simulink model "Pub_Sensor_20180704"  (R2018a)
settings: Solver=VariableStepAuto  StartTime=0.0  StopTime=inf  RelTol=1e-3
undefined symbols (not defined in the file or in its folder): D, DiscIntNeverNeededParam, G, serial, Twist
libraries: xpcutilitieslib x20, instrumentlib x9, robotlib x4, commutil2 x2, dsparch4 x1, simulink x1
settings Model: Creator=Nishida-Lab  LastModifiedBy=Nishida-Lab

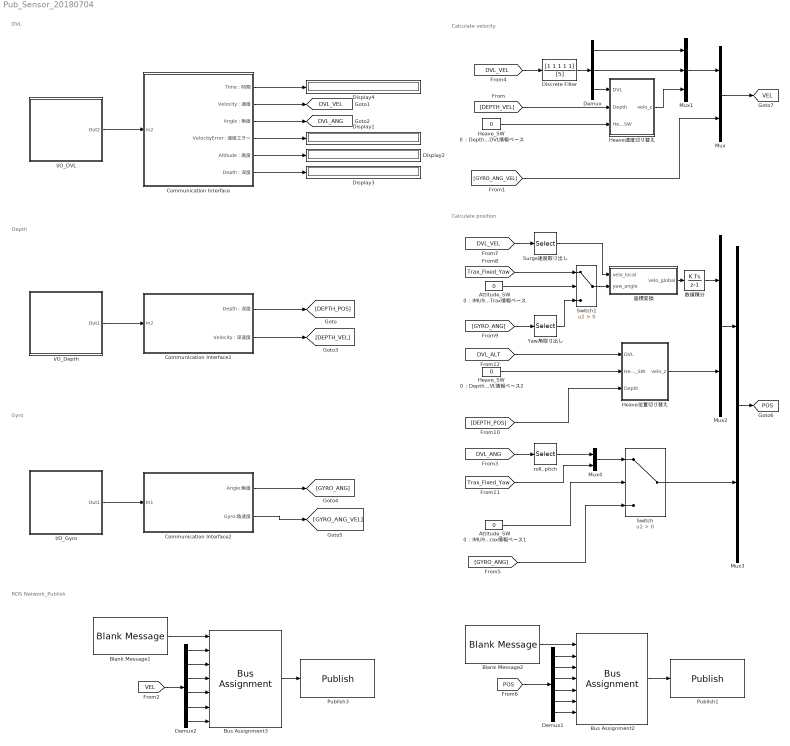
== system Pub_Sensor_20180704 ==
  note: ROS Network_Publish
  note: Gyro
  note: Depth
  note: DVL
  note: Calculate velocity
  note: Calculate position
  Attitude_SW ０：IMU9250情報ベース １：Trax情報ベース : Constant  Value=0
  Attitude_SW ０：IMU9250情報ベース １：Trax情報ベース1 : Constant  Value=0
  Blank Message1 : robotlib/Blank Message  SourceLibraryInfo=This block requires Robotics System Toolbox  messageType=geometry_msgs/TwistStamped  SampleTime=inf
      settings: SourceProductBaseCode=RO
  Blank Message2 : robotlib/Blank Message  SourceLibraryInfo=This block requires Robotics System Toolbox  messageType=geometry_msgs/TwistStamped  SampleTime=inf
      settings: SourceProductBaseCode=RO
  Bus Assignment2 : BusAssignment  AssignedSignals=Twist.Linear.X,Twist.Linear.Y,Twist.Linear.Z,Twist.Angular.X,Twist.Angular.Y,Twist.Angular.Z
  Bus Assignment3 : BusAssignment  AssignedSignals=Twist.Linear.X,Twist.Linear.Y,Twist.Linear.Z,Twist.Angular.X,Twist.Angular.Y,Twist.Angular.Z
  Communication Interface : Subsystem
  Communication Interface1 : Subsystem
  Communication Interface2 : Subsystem
  Demux : Demux  Outputs=3
  Demux1 : Demux  Outputs=6
  Demux2 : Demux  Outputs=6
  Discrete Filter : DiscreteFilter  Numerator=[1 1 1 1 1]  Denominator=[5]
  Display{1..4} (4 alike) : Display
  Heave_SW ０：Depth情報ベース １：DVL情報ベース : Constant  Value=0
  Heave_SW ０：Depth情報ベース １：DVL情報ベース2 : Constant  Value=0
  Heave位置切り替え : Subsystem
  Heave速度切り替え : Subsystem
  I/O_DVL : Subsystem
  I/O_Depth : Subsystem
  I/O_Gyro : Subsystem
  Mux{,2..4} (4 alike) : Mux  Inputs=2
  Mux1 : Mux  Inputs=3
  Publish1 : robotlib/Publish  SourceLibraryInfo=This block requires Robotics System Toolbox  topicSource=Specify your own  topic=/RT_POS  messageType=geometry_msgs/TwistStamped  messageQueueLength=1
      settings: SourceProductBaseCode=RO
  Publish3 : robotlib/Publish  SourceLibraryInfo=This block requires Robotics System Toolbox  topicSource=Specify your own  topic=/RT_VEL  messageType=geometry_msgs/TwistStamped  messageQueueLength=1
      settings: SourceProductBaseCode=RO
  Surge速度取り出し : Selector  InputPortWidth=3  IndexOptions=Index vector (dialog)  Indices=[1 2]  OutputSizes=1
  Switch : Switch  Criteria=u2 > Threshold
  Switch1 : Switch  Criteria=u2 > Threshold
  Yaw角取り出し : Selector  InputPortWidth=3  IndexOptions=Index vector (dialog)  Indices=[3]  OutputSizes=1
  "roll, pitch" : Selector  InputPortWidth=3  IndexOptions=Index vector (dialog)  Indices=[1 2]  OutputSizes=1
  座標変換 : MATLAB Function  TreatAsAtomicUnit=on
  数値積分 : DiscreteIntegrator  InitialCondition=[0 ; 0]  SampleTime=-1  ICPrevOutput=DiscIntNeverNeededParam  ICPrevScaledInput=DiscIntNeverNeededParam
  tag scope: DVL_ANG=global, DVL_VEL=global, POS=global, VEL=global
  wires:
  I/O_Depth/1(Out1) -> Communication Interface1/1(In2)
  I/O_DVL/1(Out2) -> Communication Interface/1(In2)
  Communication Interface/1(Time：時間) -> Display4/1
  Communication Interface/2(Velocity：速度) -> [DVL_VEL]
  Communication Interface/3("Angle : 角度") -> [DVL_ANG]
  Communication Interface/4(VelocityError：速度エラー) -> Display1/1
  Communication Interface/5(Altitude：高度) -> Display2/1
  Communication Interface/6(Depth：深度) -> Display3/1
  Communication Interface1/2(Velocity：深速度) -> [DEPTH_VEL]
  Communication Interface1/1(Depth：深度) -> [DEPTH_POS]
  I/O_Gyro/1(Out1) -> Communication Interface2/1(In1)
  Communication Interface2/1(Angle:角度) -> [GYRO_ANG]
  Communication Interface2/2(Gyro:角速度) -> [GYRO_ANG_VEL]
  Heave_SW ０：Depth情報ベース １：DVL情報ベース2/1 -> Heave位置切り替え/2(Heave_SW)
  [Trax_Fixed_Yaw] -> Switch1/1
  Heave速度切り替え/1(velo_z) -> Mux1/3
  Yaw角取り出し/1 -> Switch1/3
  [GYRO_ANG] -> Switch/3
  [DEPTH_POS] -> Heave位置切り替え/3(Depth)
  Heave位置切り替え/1(velo_z) -> Mux2/2
  [GYRO_ANG] -> Yaw角取り出し/1
  Mux3/1 -> [POS]
  Switch1/1 -> 座標変換/2(yaw_angle)
  [DVL_ALT] -> Heave位置切り替え/1(DVL)
  座標変換/1(velo_global) -> 数値積分/1
  Mux2/1 -> Mux3/1
  Attitude_SW ０：IMU9250情報ベース １：Trax情報ベース1/1 -> Switch/2
  "roll, pitch"/1 -> Mux4/1
  Demux/2 -> Mux1/2
  数値積分/1 -> Mux2/1
  [DVL_VEL] -> Surge速度取り出し/1
  [Trax_Fixed_Yaw] -> Mux4/2
  Attitude_SW ０：IMU9250情報ベース １：Trax情報ベース/1 -> Switch1/2
  Mux/1 -> [VEL]
  Mux1/1 -> Mux/1
  [DVL_ANG] -> "roll, pitch"/1
  Switch/1 -> Mux3/2
  Discrete Filter/1 -> Demux/1
  Demux/1 -> Mux1/1
  Surge速度取り出し/1 -> 座標変換/1(velo_local)
  Heave_SW ０：Depth情報ベース １：DVL情報ベース/1 -> Heave速度切り替え/3(HeaveSW)
  Demux/3 -> Heave速度切り替え/1(DVL)
  [GYRO_ANG_VEL] -> Mux/2
  [DEPTH_VEL] -> Heave速度切り替え/2(Depth)
  [DVL_VEL] -> Discrete Filter/1
  Mux4/1 -> Switch/1
  Bus Assignment3/1 -> Publish3/1
  Demux2/3 -> Bus Assignment3/4
  [VEL] -> Demux2/1
  Demux2/2 -> Bus Assignment3/3
  Demux2/4 -> Bus Assignment3/5
  Demux2/6 -> Bus Assignment3/7
  Demux2/5 -> Bus Assignment3/6
  Blank Message1/1 -> Bus Assignment3/1
  Demux2/1 -> Bus Assignment3/2
  Demux1/1 -> Bus Assignment2/2
  [POS] -> Demux1/1
  Demux1/3 -> Bus Assignment2/4
  Demux1/6 -> Bus Assignment2/7
  Demux1/2 -> Bus Assignment2/3
  Blank Message2/1 -> Bus Assignment2/1
  Demux1/4 -> Bus Assignment2/5
  Bus Assignment2/1 -> Publish1/1
  Demux1/5 -> Bus Assignment2/6

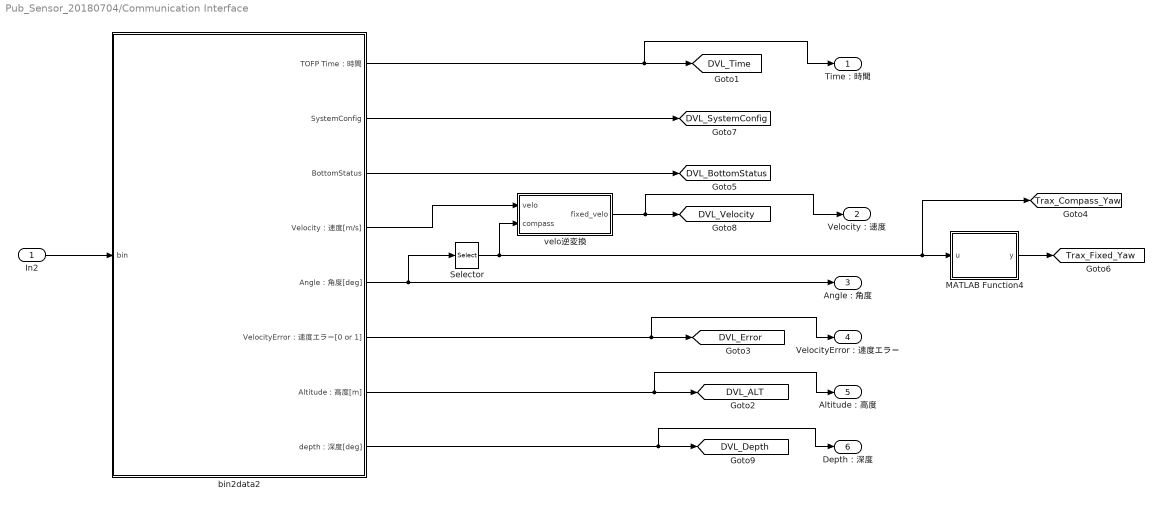
== system Pub_Sensor_20180704/Communication Interface ==
  In2 : Inport
  MATLAB Function4 : MATLAB Function  TreatAsAtomicUnit=on
  Selector : Selector  InputPortWidth=3  IndexOptions=Index vector (dialog)  Indices=[3]  OutputSizes=1
  bin2data2 : Subsystem
  velo逆変換 : Subsystem
  Time：時間 : Outport
  Velocity：速度 : Outport  Port=2
  "Angle : 角度" : Outport  Port=3
  VelocityError：速度エラー : Outport  Port=4
  Altitude：高度 : Outport  Port=5
  Depth：深度 : Outport  Port=6
  tag scope: DVL_ALT=global, DVL_BottomStatus=global, DVL_Depth=global, DVL_Error=global, DVL_SystemConfig=global, DVL_Time=global, DVL_Velocity=global, Trax_Compass_Yaw=global, Trax_Fixed_Yaw=global
  wires:
  velo逆変換/1(fixed_velo) -> Velocity：速度/1, [DVL_Velocity]
  bin2data2/5(Angle：角度[deg]) -> Selector/1, "Angle : 角度"/1
  bin2data2/3(BottomStatus) -> [DVL_BottomStatus]
  bin2data2/8(depth：深度[deg]) -> Depth：深度/1, [DVL_Depth]
  In2/1 -> bin2data2/1(bin)
  MATLAB Function4/1(y) -> [Trax_Fixed_Yaw]
  bin2data2/7(Altitude：高度[m]) -> [DVL_ALT], Altitude：高度/1
  bin2data2/6(VelocityError：速度エラー[0 or 1]) -> [DVL_Error], VelocityError：速度エラー/1
  bin2data2/1(TOFP Time：時間) -> Time：時間/1, [DVL_Time]
  bin2data2/2(SystemConfig) -> [DVL_SystemConfig]
  bin2data2/4(Velocity：速度[m/s]) -> velo逆変換/1(velo)
  Selector/1 -> [Trax_Compass_Yaw], MATLAB Function4/1(u), velo逆変換/2(compass)

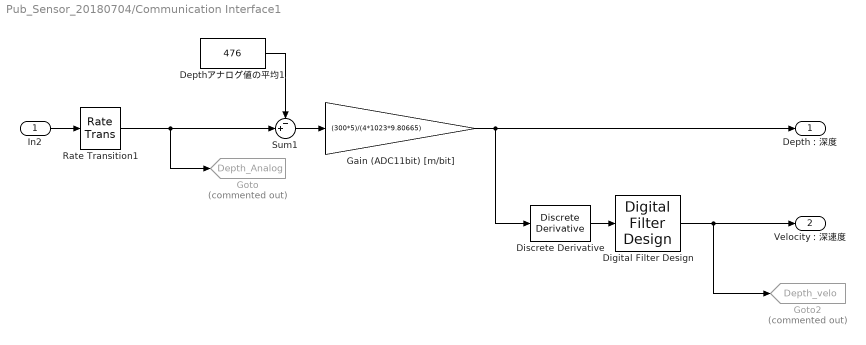
== system Pub_Sensor_20180704/Communication Interface1 ==
  In2 : Inport
  Depthアナログ値の平均1 : Constant  Value=476
  Digital Filter Design : dsparch4/Digital Filter Design  mwdsp_browser_bugfix_var=off
  Discrete Derivative : simulink/Discrete/Discrete Derivative  gainval=1.0  ICPrevScaledInput=0.0  InputProcessing=Inherited  OutMin=[]  OutMax=[]  OutDataType=fixdt(1, 16)  OutScaling=2^-10  DoSatur=off
  Gain (ADC11bit) [m/bit] : Gain  Gain=(300*5)/(4*1023*9.80665)
  Goto : Goto  Commented=on  GotoTag=Depth_Analog  TagVisibility=global
  Goto2 : Goto  Commented=on  GotoTag=Depth_velo  TagVisibility=global
  Rate Transition1 : RateTransition  OutPortSampleTime=0.1
  Sum1 : Sum  Inputs=-+|
  Depth：深度 : Outport
  Velocity：深速度 : Outport  Port=2
  wires:
  Digital Filter Design/1 -> Goto2/1, Velocity：深速度/1
  In2/1 -> Rate Transition1/1
  Gain (ADC11bit) [m/bit]/1 -> Discrete Derivative/1, Depth：深度/1
  Sum1/1 -> Gain (ADC11bit) [m/bit]/1
  Depthアナログ値の平均1/1 -> Sum1/1
  Rate Transition1/1 -> Goto/1, Sum1/2
  Discrete Derivative/1 -> Digital Filter Design/1

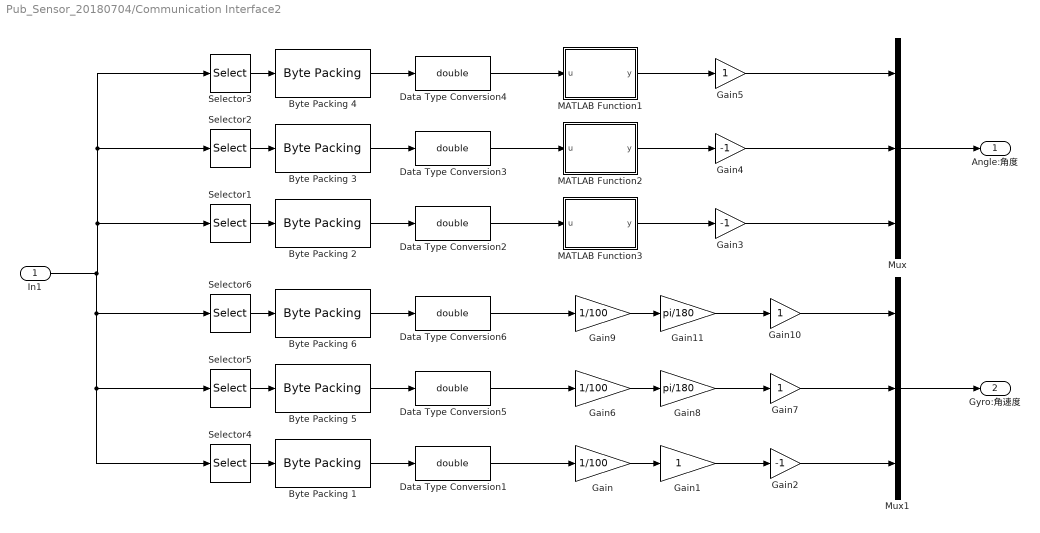
== system Pub_Sensor_20180704/Communication Interface2 ==
  In1 : Inport
  Byte Packing {1..6} (6 alike) : xpcutilitieslib/Byte Packing 
  Data Type Conversion{1..6} (6 alike) : DataTypeConversion  OutDataTypeStr=double
  Gain : Gain  Gain=1/100
  Gain{1,5,7,10} (4 alike) : Gain
  Gain11 : Gain  Gain=pi/180
  Gain2 : Gain  Gain=-1
  Gain3 : Gain  Gain=-1
  Gain4 : Gain  Gain=-1
  Gain6 : Gain  Gain=1/100
  Gain8 : Gain  Gain=pi/180
  Gain9 : Gain  Gain=1/100
  MATLAB Function1 : MATLAB Function  TreatAsAtomicUnit=on
  MATLAB Function2 : MATLAB Function  TreatAsAtomicUnit=on
  MATLAB Function3 : MATLAB Function  TreatAsAtomicUnit=on
  Mux : Mux  Inputs=3
  Mux1 : Mux  Inputs=3
  Selector1 : Selector  InputPortWidth=12  IndexOptions=Index vector (dialog)  Indices=[2 1]  OutputSizes=1
  Selector2 : Selector  InputPortWidth=12  IndexOptions=Index vector (dialog)  Indices=[4 3]  OutputSizes=1
  Selector3 : Selector  InputPortWidth=12  IndexOptions=Index vector (dialog)  Indices=[6 5]  OutputSizes=1
  Selector4 : Selector  InputPortWidth=12  IndexOptions=Index vector (dialog)  Indices=[8 7]  OutputSizes=1
  Selector5 : Selector  InputPortWidth=12  IndexOptions=Index vector (dialog)  Indices=[10 9]  OutputSizes=1
  Selector6 : Selector  InputPortWidth=12  IndexOptions=Index vector (dialog)  Indices=[12 11]  OutputSizes=1
  Angle:角度 : Outport
  Gyro:角速度 : Outport  Port=2
  wires:
  In1/1 -> Selector2/1, Selector3/1, Selector1/1, Selector4/1, Selector5/1, Selector6/1
  Gain/1 -> Gain1/1
  Byte Packing 1/1 -> Data Type Conversion1/1
  MATLAB Function3/1(y) -> Gain3/1
  Data Type Conversion4/1 -> MATLAB Function1/1(u)
  Gain3/1 -> Mux/3
  Selector6/1 -> Byte Packing 6/1
  Selector2/1 -> Byte Packing 3/1
  Gain6/1 -> Gain8/1
  MATLAB Function2/1(y) -> Gain4/1
  Gain8/1 -> Gain7/1
  Data Type Conversion1/1 -> Gain/1
  Selector4/1 -> Byte Packing 1/1
  Gain4/1 -> Mux/2
  Gain2/1 -> Mux1/3
  Selector3/1 -> Byte Packing 4/1
  Data Type Conversion5/1 -> Gain6/1
  Data Type Conversion3/1 -> MATLAB Function2/1(u)
  Gain10/1 -> Mux1/1
  Data Type Conversion6/1 -> Gain9/1
  Byte Packing 5/1 -> Data Type Conversion5/1
  Gain9/1 -> Gain11/1
  Gain5/1 -> Mux/1
  Gain11/1 -> Gain10/1
  Data Type Conversion2/1 -> MATLAB Function3/1(u)
  Byte Packing 6/1 -> Data Type Conversion6/1
  MATLAB Function1/1(y) -> Gain5/1
  Gain7/1 -> Mux1/2
  Mux/1 -> Angle:角度/1
  Gain1/1 -> Gain2/1
  Byte Packing 3/1 -> Data Type Conversion3/1
  Byte Packing 2/1 -> Data Type Conversion2/1
  Byte Packing 4/1 -> Data Type Conversion4/1
  Selector5/1 -> Byte Packing 5/1
  Mux1/1 -> Gyro:角速度/1
  Selector1/1 -> Byte Packing 2/1

== system Pub_Sensor_20180704/Heave位置切り替え ==
  DVL : Inport
  Heave_SW : Inport  Port=2
  Depth : Inport  Port=3
  Switch : Switch  Criteria=u2 > Threshold
  velo_z : Outport
  wires:
  Depth/1 -> Switch/3
  DVL/1 -> Switch/1
  Heave_SW/1 -> Switch/2
  Switch/1 -> velo_z/1

== system Pub_Sensor_20180704/Heave速度切り替え ==
  DVL : Inport
  Depth : Inport  Port=2
  HeaveSW : Inport  Port=3
  Switch : Switch  Criteria=u2 > Threshold
  velo_z : Outport
  wires:
  Depth/1 -> Switch/3
  DVL/1 -> Switch/1
  HeaveSW/1 -> Switch/2
  Switch/1 -> velo_z/1

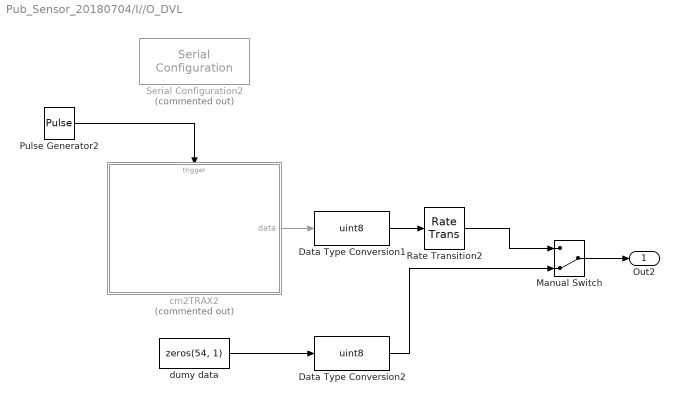
== system Pub_Sensor_20180704/I//O_DVL ==
  Data Type Conversion1 : DataTypeConversion  OutDataTypeStr=uint8
  Data Type Conversion2 : DataTypeConversion  OutDataTypeStr=uint8
  Manual Switch : ManualSwitch  CurrentSetting=0
  Pulse Generator2 : DiscretePulseGenerator  PulseType=Time based  Period=0.2  PulseWidth=50
  Rate Transition2 : RateTransition  OutPortSampleTime=0.1
  Serial Configuration2 : instrumentlib/Serial Configuration  Priority=-200000  Commented=on  ComPortMenu=<Please select a port...>  ComPort=COM7  ObjConstructor=serial('COM7');  BaudRate=115200  DataBits=8  Parity=none  StopBits=1  FlowControl=none  Timeout=10  ByteOrder=LittleEndian
  cm2TRAX2 : Stateflow chart  Commented=on  TreatAsAtomicUnit=on
  dumy data : Constant  Value=zeros(54, 1)
  Out2 : Outport
  wires:
  cm2TRAX2/1(data) -> Data Type Conversion1/1
  Data Type Conversion2/1 -> Manual Switch/2
  Rate Transition2/1 -> Manual Switch/1
  Data Type Conversion1/1 -> Rate Transition2/1
  Manual Switch/1 -> Out2/1
  dumy data/1 -> Data Type Conversion2/1
  Pulse Generator2/1 -> cm2TRAX2/Trigger

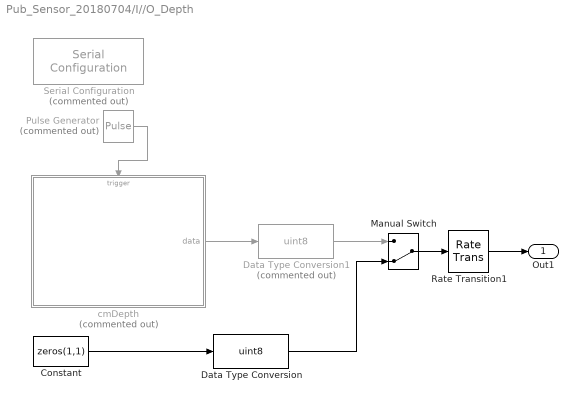
== system Pub_Sensor_20180704/I//O_Depth ==
  Constant : Constant  Value=zeros(1,1)  VectorParams1D=off
  Data Type Conversion : DataTypeConversion  OutDataTypeStr=uint8
  Data Type Conversion1 : DataTypeConversion  Commented=on  OutDataTypeStr=uint8
  Manual Switch : ManualSwitch  CurrentSetting=0
  Pulse Generator : DiscretePulseGenerator  Commented=on  PulseType=Time based  Period=0.1  PulseWidth=50
  Rate Transition1 : RateTransition  OutPortSampleTime=0.1
  Serial Configuration : instrumentlib/Serial Configuration  Priority=-200000  Commented=on  ComPortMenu=<Please select a port...>  ComPort=COM21  ObjConstructor=serial('COM21');  BaudRate=115200  DataBits=8  Parity=none  StopBits=1  FlowControl=none  Timeout=10  ByteOrder=LittleEndian
  cmDepth : Stateflow chart  Commented=on  TreatAsAtomicUnit=on
  Out1 : Outport
  wires:
  Pulse Generator/1 -> cmDepth/Trigger
  Constant/1 -> Data Type Conversion/1
  Data Type Conversion/1 -> Manual Switch/2
  Manual Switch/1 -> Rate Transition1/1
  Rate Transition1/1 -> Out1/1
  Data Type Conversion1/1 -> Manual Switch/1
  cmDepth/1(data) -> Data Type Conversion1/1

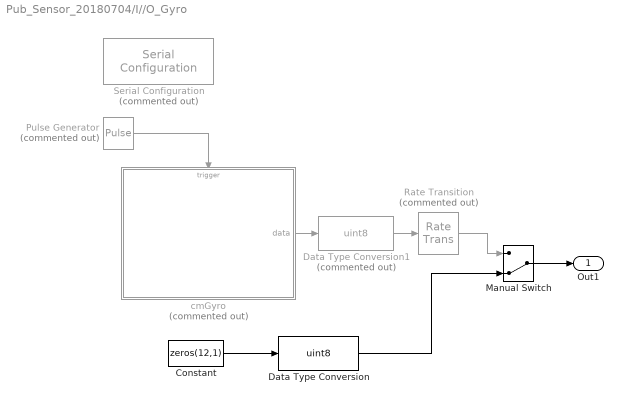
== system Pub_Sensor_20180704/I//O_Gyro ==
  Constant : Constant  Value=zeros(12,1)
  Data Type Conversion : DataTypeConversion  OutDataTypeStr=uint8
  Data Type Conversion1 : DataTypeConversion  Commented=on  OutDataTypeStr=uint8
  Manual Switch : ManualSwitch  CurrentSetting=0
  Pulse Generator : DiscretePulseGenerator  Commented=on  PulseType=Time based  Period=0.1  PulseWidth=50
  Rate Transition : RateTransition  Commented=on  OutPortSampleTime=0.1
  Serial Configuration : instrumentlib/Serial Configuration  Priority=-200000  Commented=on  ComPortMenu=<Please select a port...>  ComPort=COM14  ObjConstructor=serial('COM14');  BaudRate=115200  DataBits=8  Parity=none  StopBits=1  FlowControl=none  Timeout=10  ByteOrder=LittleEndian
  cmGyro : Stateflow chart  Commented=on  TreatAsAtomicUnit=on
  Out1 : Outport
  wires:
  cmGyro/1(data) -> Data Type Conversion1/1
  Pulse Generator/1 -> cmGyro/Trigger
  Data Type Conversion1/1 -> Rate Transition/1
  Data Type Conversion/1 -> Manual Switch/2
  Manual Switch/1 -> Out1/1
  Constant/1 -> Data Type Conversion/1
  Rate Transition/1 -> Manual Switch/1

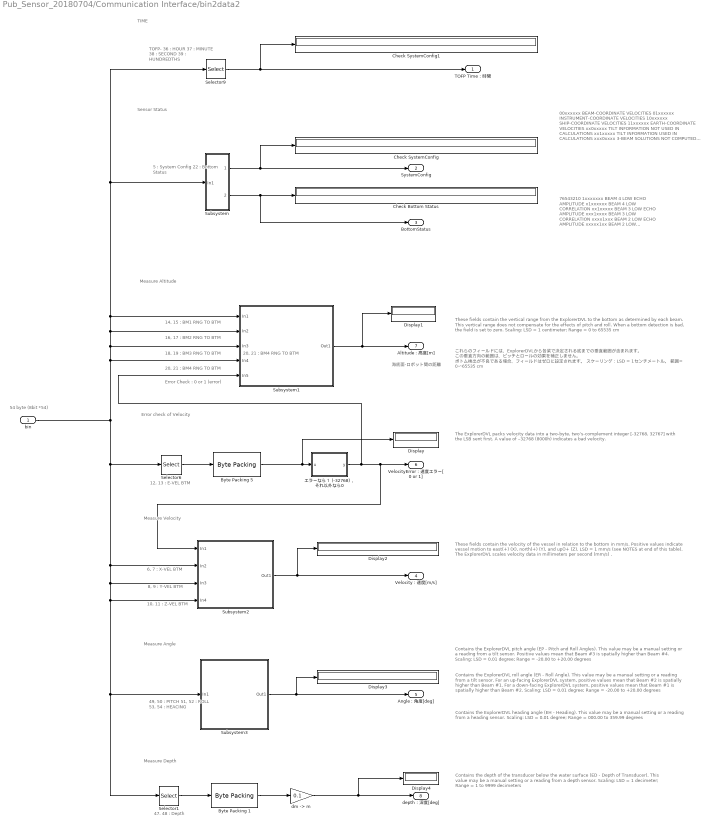
== system Pub_Sensor_20180704/Communication Interface/bin2data2 ==
  note: Contains the depth of the transducer below the water surface (ED - Depth of Transducer).
      | This value may be a manual setting or a reading from a depth sensor.
      | Scaling: LSD = 1 decimeter; Range = 1 to 9999 decimeters
  note: 54 byte (8bit *54)
  note: Contains the ExplorerDVL heading angle (EH - Heading). This value may be a manual setting or a reading from a heading sensor.
      | Scaling: LSD = 0.01 degree; Range = 000.00 to 359.99 degrees
  note: Contains the ExplorerDVL roll angle (ER - Roll Angle). This value may be a manual setting or a reading from a tilt sensor. For an up-facing ExplorerDVL system, positive values mean that Beam #2 is spatially higher than Beam #1. For a down-facing ExplorerDVL system, positive values mean that Beam #1 is spatially higher than Beam #2.
      | Scaling: LSD = 0.01 degree; Range = -20.00 to +20.00 degrees
  note: Contains the ExplorerDVL pitch angle (EP - Pitch and Roll Angles). This value may be a manual setting or a reading from a tilt sensor. Positive values mean that Beam #3 is spatially higher than Beam #4.
      | Scaling: LSD = 0.01 degree; Range = -20.00 to +20.00 degrees
  note: The ExplorerDVL packs velocity data into a two-byte, two’s-complement integer [-32768, 32767]
      | with the LSB sent first.
      | A value of –32768 (8000h) indicates a bad velocity.
  note: These fields contain the velocity of the vessel in relation to the bottom in mm/s. Positive
      | values indicate vessel motion to east(+) (X), north(+) (Y), and up()+ (Z). LSD = 1 mm/s (see NOTES at
      | end of this table).
      | The ExplorerDVL scales velocity data in millimeters per second (mm/s) .
  note: これらのフィールドには、ExplorerDVLから各梁で決定される底までの垂直範囲が含まれます。
      | この垂直方向の範囲は、ピッチとロールの効果を補正しません。
      | ボトム検出が不良である場合、フィールドはゼロに設定されます。
      | スケーリング：LSD = 1センチメートル。 範囲= 0〜65535 cm
  note: 海底面-ロボット間の距離
  note: These fields contain the vertical range from the ExplorerDVL to the bottom as determined by each beam.
      | This vertical range does not compensate for the effects of pitch and roll.
      | When a bottom detection is bad, the field is set to zero.
      | Scaling: LSD = 1 centimeter; Range = 0 to 65535 cm
  note: Measure Altitude
  note: 5 : System Config
      | 22 : Bottom Status
  note: 76543210
      | 1xxxxxxx BEAM 4 LOW ECHO AMPLITUDE
      | x1xxxxxx BEAM 4 LOW CORRELATION
      | xx1xxxxx BEAM 3 LOW ECHO AMPLITUDE
      | xxx1xxxx BEAM 3 LOW CORRELATION
      | xxxx1xxx BEAM 2 LOW ECHO AMPLITUDE
      | xxxxx1xx BEAM 2 LOW CORRELATION
      | xxxxxx1x BEAM 1 LOW ECHO AMPLITUDE
      | xxxxxxx1 BEAM 1 LOW CORRELATION
  note: 00xxxxxx BEAM-COORDINATE VELOCITIES
      | 01xxxxxx INSTRUMENT-COORDINATE VELOCITIES
      | 10xxxxxx SHIP-COORDINATE VELOCITIES
      | 11xxxxxx EARTH-COORDINATE VELOCITIES
      | xx0xxxxx TILT INFORMATION NOT USED IN CALCULATIONS
      | xx1xxxxx TILT INFORMATION USED IN CALCULATIONS
      | xxx0xxxx 3-BEAM SOLUTIONS NOT COMPUTED
      | xxx1xxxx 3-BEAM SOLUTIONS COMPUTED
      | xxxxx001 150-kHz ExplorerDVL
      | xxxxx010 300-kHz ExplorerDVL
      | xxxxx011 600-kHz ExplorerDVL
      | xxxxx100 1200-kHz ExplorerDVL
  note: TIME
  note: 12, 13 : E-VEL BTM
  note: TOFP-
      | 36 : HOUR
      | 37 : MINUTE
      | 38 : SECOND
      | 39 : HUNDREDTHS
  note: Sensor Status
  note: 14, 15 : BM1 RNG TO BTM
  note: 16, 17 : BM2 RNG TO BTM
  note: 18, 19 : BM3 RNG TO BTM
  note: 20, 21 : BM4 RNG TO BTM
  note: 20, 21 : BM4 RNG TO BTM
  note: Error Check : 0 or 1 (error)
  note: Error check of Velocity
  note: Measure Velocity
  note: 6, 7 : X-VEL BTM
  note: 8, 9 : Y-VEL BTM
  note: 10, 11 : Z-VEL BTM
  note: 49, 50 : PITCH
      | 51, 52 : ROLL
      | 53, 54 : HEACING
  note: Measure Angle
  note: Measure Depth
  note: 47. 48 : Depth
  bin : Inport
  Byte Packing 1 : xpcutilitieslib/Byte Packing   MaskPackedDataType=int16  MaskUnpackedDataTypes={'uint8'}  MaskAlignment=2
  Byte Packing 5 : xpcutilitieslib/Byte Packing   MaskPackedDataType=int16  MaskUnpackedDataTypes={'uint8'}  MaskAlignment=2
  Check Bottom Status : Display
  Check SystemConfig : Display
  Check SystemConfig1 : Display
  Display{,1..4} (5 alike) : Display
  Selector1 : Selector  InputPortWidth=54  IndexOptions=Index vector (dialog)  Indices=[47 48]  OutputSizes=1
  Selector6 : Selector  InputPortWidth=54  IndexOptions=Index vector (dialog)  Indices=[12 13]  OutputSizes=1
  Selector9 : Selector  InputPortWidth=54  IndexOptions=Index vector (dialog)  Indices=[36 37 38 39]  OutputSizes=1
  Subsystem : Subsystem
  Subsystem1 : Subsystem
  Subsystem2 : Subsystem
  Subsystem3 : Subsystem
  "dm -> m" : Gain  Gain=0.1  OutDataTypeStr=double
  エラーなら１ (-32768)， それ以外なら0 : MATLAB Function  TreatAsAtomicUnit=on
  TOFP Time：時間 : Outport
  SystemConfig : Outport  Port=2
  BottomStatus : Outport  Port=3
  Velocity：速度[m/s] : Outport  Port=4
  Angle：角度[deg] : Outport  Port=5
  VelocityError：速度エラー[0 or 1] : Outport  Port=6
  Altitude：高度[m] : Outport  Port=7
  depth：深度[deg] : Outport  Port=8
  wires:
  Selector6/1 -> Byte Packing 5/1
  Byte Packing 5/1 -> Display/1, エラーなら１ (-32768)， それ以外なら0/1(u)
  Selector9/1 -> Check SystemConfig1/1, TOFP Time：時間/1
  エラーなら１ (-32768)， それ以外なら0/1(y) -> Subsystem1/5(In5), Subsystem2/1(In1), VelocityError：速度エラー[0 or 1]/1
  bin/1 -> Subsystem1/2(In2), Selector9/1, Subsystem/1(In1), Subsystem1/1(In1), Subsystem1/3(In3), Subsystem1/4(In4), Subsystem2/3(In3), Selector1/1, Subsystem3/1(In1), Subsystem2/4(In4), Subsystem2/2(In2), Selector6/1
  Subsystem/1(Out1) -> SystemConfig/1, Check SystemConfig/1
  Subsystem/2(Out2) -> BottomStatus/1, Check Bottom Status/1
  Subsystem1/1(Out1) -> Display1/1, Altitude：高度[m]/1
  Subsystem2/1(Out1) -> Display2/1, Velocity：速度[m/s]/1
  Subsystem3/1(Out1) -> Display3/1, Angle：角度[deg]/1
  Selector1/1 -> Byte Packing 1/1
  Byte Packing 1/1 -> "dm -> m"/1
  "dm -> m"/1 -> depth：深度[deg]/1, Display4/1

== system Pub_Sensor_20180704/Communication Interface/velo逆変換 ==
  velo : Inport
  compass : Inport  Port=2
  MATLAB Function : MATLAB Function  TreatAsAtomicUnit=on
  fixed_velo : Outport
  wires:
  velo/1 -> MATLAB Function/1(velo)
  compass/1 -> MATLAB Function/2(angle)
  MATLAB Function/1(y) -> fixed_velo/1

== system Pub_Sensor_20180704/I//O_DVL/cm2TRAX2/recieve.recieve_data ==
  f : TriggerPort  TriggerType=function-call  VariantControl=Variant
      settings: CopyFcn=Stateflow.SLINSF.SimulinkMan.removeBlockPreDeleteFcn  PreDeleteFcn=Stateflow.SLINSF.SimulinkMan.unsafePredeleteFcn
  Serial Receive : instrumentlib/Serial Receive  ComPortMenu=<Please select a port...>  ComPort=COM7  ObjConstructor=serial('COM7');  Header=CS<  Terminator=<none>  DataSize=54  DataType=uint8  EnableBlockingMode=off  ActionDataUnavailable=Output last received value  CustomValue=0  SampleTime=-1
  data : Outport  OutDataTypeStr=uint8  PortDimensions=54
  wires:
  Serial Receive/1 -> data/1

== system Pub_Sensor_20180704/I//O_DVL/cm2TRAX2/send.send_q ==
  f : TriggerPort  TriggerType=function-call  VariantControl=Variant
      settings: CopyFcn=Stateflow.SLINSF.SimulinkMan.removeBlockPreDeleteFcn  PreDeleteFcn=Stateflow.SLINSF.SimulinkMan.unsafePredeleteFcn
  Constant1 : Constant  Value=67  OutDataTypeStr=uint8
  Constant2 : Constant  Value=13  OutDataTypeStr=uint8
  Constant3 : Constant  Value=10  OutDataTypeStr=uint8
  Constant4 : Constant  Value=83  OutDataTypeStr=uint8
  Mux : Mux
  Serial Send : instrumentlib/Serial Send  ComPortMenu=<Please select a port...>  ComPort=COM7  ObjConstructor=serial('COM7');  Terminator=<none>  EnableBlockingMode=off
  wires:
  Mux/1 -> Serial Send/1
  Constant2/1 -> Mux/3
  Constant3/1 -> Mux/4
  Constant4/1 -> Mux/2
  Constant1/1 -> Mux/1

== system Pub_Sensor_20180704/I//O_Depth/cmDepth/recieve.recieve_data ==
  f : TriggerPort  TriggerType=function-call  VariantControl=Variant
      settings: CopyFcn=Stateflow.SLINSF.SimulinkMan.removeBlockPreDeleteFcn  PreDeleteFcn=Stateflow.SLINSF.SimulinkMan.unsafePredeleteFcn
  Serial Receive : instrumentlib/Serial Receive  ComPortMenu=<Please select a port...>  ComPort=COM21  ObjConstructor=serial('COM21');  Header=D:  Terminator=<none>  DataSize=1  DataType=int16  EnableBlockingMode=off  ActionDataUnavailable=Output last received value  CustomValue=0  SampleTime=-1
  data : Outport  OutDataTypeStr=int16  PortDimensions=1
  wires:
  Serial Receive/1 -> data/1

== system Pub_Sensor_20180704/I//O_Depth/cmDepth/send.send_q ==
  f : TriggerPort  TriggerType=function-call  VariantControl=Variant
      settings: CopyFcn=Stateflow.SLINSF.SimulinkMan.removeBlockPreDeleteFcn  PreDeleteFcn=Stateflow.SLINSF.SimulinkMan.unsafePredeleteFcn
  'd'の10進数表現 : Constant  Value=100  OutDataTypeStr=uint8
  Serial Send : instrumentlib/Serial Send  ComPortMenu=<Please select a port...>  ComPort=COM21  ObjConstructor=serial('COM21');  Terminator=<none>  EnableBlockingMode=on
  wires:
  'd'の10進数表現/1 -> Serial Send/1

== system Pub_Sensor_20180704/I//O_Gyro/cmGyro/recieve.recieve_data ==
  f : TriggerPort  TriggerType=function-call  VariantControl=Variant
      settings: CopyFcn=Stateflow.SLINSF.SimulinkMan.removeBlockPreDeleteFcn  PreDeleteFcn=Stateflow.SLINSF.SimulinkMan.unsafePredeleteFcn
  Serial Receive : instrumentlib/Serial Receive  ComPortMenu=<Please select a port...>  ComPort=COM14  ObjConstructor=serial('COM14');  Header=G:  Terminator=<none>  DataSize=12  DataType=uint8  EnableBlockingMode=off  ActionDataUnavailable=Output last received value  CustomValue=0  SampleTime=-1
  data : Outport  OutDataTypeStr=uint8  PortDimensions=12
  wires:
  Serial Receive/1 -> data/1

== system Pub_Sensor_20180704/I//O_Gyro/cmGyro/send.send_q ==
  f : TriggerPort  TriggerType=function-call  VariantControl=Variant
      settings: CopyFcn=Stateflow.SLINSF.SimulinkMan.removeBlockPreDeleteFcn  PreDeleteFcn=Stateflow.SLINSF.SimulinkMan.unsafePredeleteFcn
  'g'の10進数表現 : Constant  Value=103  OutDataTypeStr=uint8
  Serial Send : instrumentlib/Serial Send  ComPortMenu=<Please select a port...>  ComPort=COM14  ObjConstructor=serial('COM14');  Terminator=<none>  EnableBlockingMode=off
  wires:
  'g'の10進数表現/1 -> Serial Send/1

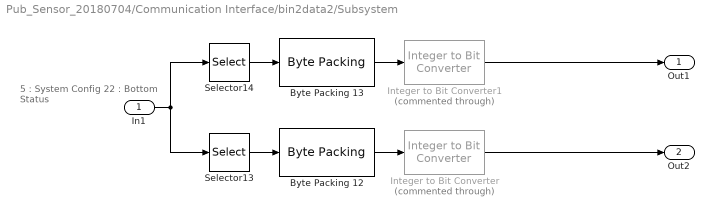
== system Pub_Sensor_20180704/Communication Interface/bin2data2/Subsystem ==
  note: 5 : System Config
      | 22 : Bottom Status
  In1 : Inport
  Byte Packing 12 : xpcutilitieslib/Byte Packing   MaskPackedDataType=uint8  MaskUnpackedDataTypes={'uint8'}  MaskAlignment=1
  Byte Packing 13 : xpcutilitieslib/Byte Packing   MaskPackedDataType=uint8  MaskUnpackedDataTypes={'uint8'}  MaskAlignment=1
  Integer to Bit Converter : commutil2/Integer to Bit Converter  Commented=through  nbits=8  signedInputValues=Unsigned  bitOrder=MSB first  outDtype=Inherit via internal rule
  Integer to Bit Converter1 : commutil2/Integer to Bit Converter  Commented=through  nbits=8  signedInputValues=Unsigned  bitOrder=MSB first  outDtype=Inherit via internal rule
  Selector13 : Selector  InputPortWidth=54  IndexOptions=Index vector (dialog)  Indices=[22]  OutputSizes=1
  Selector14 : Selector  InputPortWidth=54  IndexOptions=Index vector (dialog)  Indices=[5]  OutputSizes=1
  Out1 : Outport
  Out2 : Outport  Port=2
  wires:
  Integer to Bit Converter/1 -> Out2/1
  Selector13/1 -> Byte Packing 12/1
  In1/1 -> Selector13/1, Selector14/1
  Byte Packing 13/1 -> Integer to Bit Converter1/1
  Integer to Bit Converter1/1 -> Out1/1
  Selector14/1 -> Byte Packing 13/1
  Byte Packing 12/1 -> Integer to Bit Converter/1

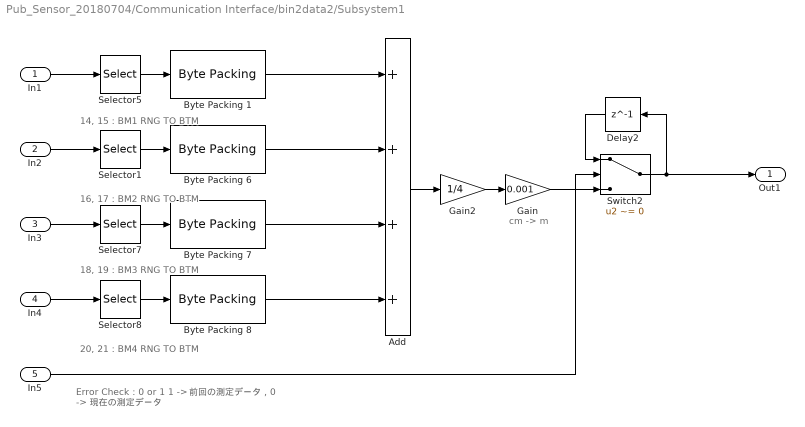
== system Pub_Sensor_20180704/Communication Interface/bin2data2/Subsystem1 ==
  note: cm -> m
  note: 14, 15 : BM1 RNG TO BTM
  note: 16, 17 : BM2 RNG TO BTM
  note: 18, 19 : BM3 RNG TO BTM
  note: 20, 21 : BM4 RNG TO BTM
  note: Error Check : 0 or 1
      | 1 -> 前回の測定データ，0 -> 現在の測定データ
  In1 : Inport
  In2 : Inport  Port=2
  In3 : Inport  Port=3
  In4 : Inport  Port=4
  In5 : Inport  Port=5
  Add : Sum  Inputs=++++
  Byte Packing {1,6..8} (4 alike) : xpcutilitieslib/Byte Packing   MaskPackedDataType=int16  MaskUnpackedDataTypes={'uint8'}  MaskAlignment=2
  Delay2 : Delay  DelayLength=1  InitialCondition=0
  Gain : Gain  Gain=0.001  OutDataTypeStr=double
  Gain2 : Gain  Gain=1/4  OutDataTypeStr=double
  Selector1 : Selector  InputPortWidth=54  IndexOptions=Index vector (dialog)  Indices=[16 17]  OutputSizes=1
  Selector5 : Selector  InputPortWidth=54  IndexOptions=Index vector (dialog)  Indices=[14 15]  OutputSizes=1
  Selector7 : Selector  InputPortWidth=54  IndexOptions=Index vector (dialog)  Indices=[18 19]  OutputSizes=1
  Selector8 : Selector  InputPortWidth=54  IndexOptions=Index vector (dialog)  Indices=[20 21]  OutputSizes=1
  Switch2 : Switch  Criteria=u2 ~= 0
  Out1 : Outport
  wires:
  Switch2/1 -> Out1/1, Delay2/1
  Gain2/1 -> Gain/1
  Byte Packing 7/1 -> Add/3
  Selector5/1 -> Byte Packing 1/1
  Selector8/1 -> Byte Packing 8/1
  Byte Packing 1/1 -> Add/1
  Selector7/1 -> Byte Packing 7/1
  Gain/1 -> Switch2/3
  Selector1/1 -> Byte Packing 6/1
  Byte Packing 8/1 -> Add/4
  Byte Packing 6/1 -> Add/2
  Delay2/1 -> Switch2/1
  In5/1 -> Switch2/2
  In3/1 -> Selector7/1
  Add/1 -> Gain2/1
  In1/1 -> Selector5/1
  In4/1 -> Selector8/1
  In2/1 -> Selector1/1

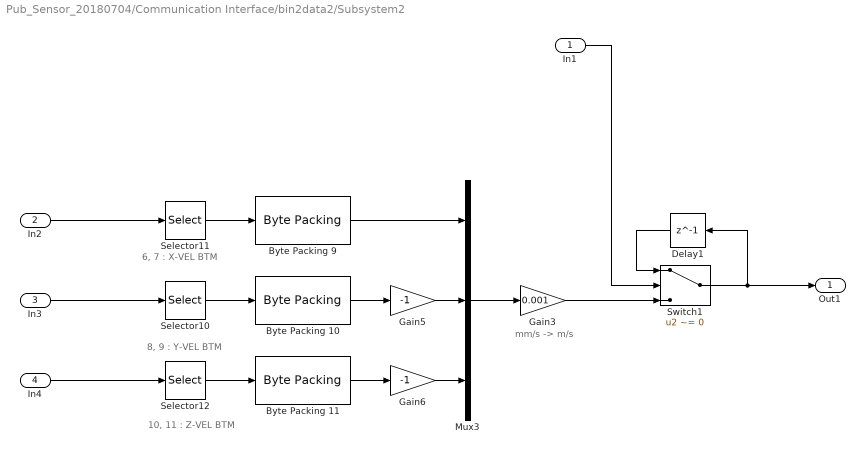
== system Pub_Sensor_20180704/Communication Interface/bin2data2/Subsystem2 ==
  note: mm/s -> m/s
  note: 6, 7 : X-VEL BTM
  note: 8, 9 : Y-VEL BTM
  note: 10, 11 : Z-VEL BTM
  In1 : Inport
  In2 : Inport  Port=2
  In3 : Inport  Port=3
  In4 : Inport  Port=4
  Byte Packing 10 : xpcutilitieslib/Byte Packing   MaskPackedDataType=int16  MaskUnpackedDataTypes={'uint8'}  MaskAlignment=2
  Byte Packing 11 : xpcutilitieslib/Byte Packing   MaskPackedDataType=int16  MaskUnpackedDataTypes={'uint8'}  MaskAlignment=2
  Byte Packing 9 : xpcutilitieslib/Byte Packing   MaskPackedDataType=int16  MaskUnpackedDataTypes={'uint8'}  MaskAlignment=2
  Delay1 : Delay  DelayLength=1  InitialCondition=0
  Gain3 : Gain  Gain=0.001  OutDataTypeStr=double
  Gain5 : Gain  Gain=-1  OutDataTypeStr=int16
  Gain6 : Gain  Gain=-1  OutDataTypeStr=int16
  Mux3 : Mux  Inputs=3
  Selector10 : Selector  InputPortWidth=54  IndexOptions=Index vector (dialog)  Indices=[8 9]  OutputSizes=1
  Selector11 : Selector  InputPortWidth=54  IndexOptions=Index vector (dialog)  Indices=[6 7]  OutputSizes=1
  Selector12 : Selector  InputPortWidth=54  IndexOptions=Index vector (dialog)  Indices=[10 11]  OutputSizes=1
  Switch1 : Switch  Criteria=u2 ~= 0  Threshold=-32767
  Out1 : Outport
  wires:
  Byte Packing 9/1 -> Mux3/1
  Gain5/1 -> Mux3/2
  Switch1/1 -> Out1/1, Delay1/1
  Selector10/1 -> Byte Packing 10/1
  Mux3/1 -> Gain3/1
  Selector11/1 -> Byte Packing 9/1
  In2/1 -> Selector11/1
  Selector12/1 -> Byte Packing 11/1
  Byte Packing 11/1 -> Gain6/1
  Gain3/1 -> Switch1/3
  Byte Packing 10/1 -> Gain5/1
  Gain6/1 -> Mux3/3
  Delay1/1 -> Switch1/1
  In3/1 -> Selector10/1
  In4/1 -> Selector12/1
  In1/1 -> Switch1/2

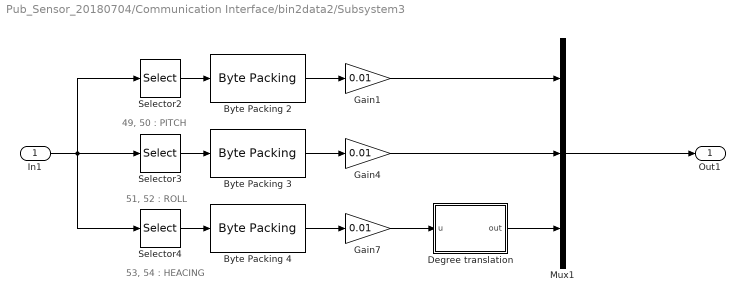
== system Pub_Sensor_20180704/Communication Interface/bin2data2/Subsystem3 ==
  note: 49, 50 : PITCH
  note: 51, 52 : ROLL
  note: 53, 54 : HEACING
  In1 : Inport
  Byte Packing 2 : xpcutilitieslib/Byte Packing   MaskPackedDataType=int16  MaskUnpackedDataTypes={'uint8'}  MaskAlignment=2
  Byte Packing 3 : xpcutilitieslib/Byte Packing   MaskPackedDataType=int16  MaskUnpackedDataTypes={'uint8'}  MaskAlignment=2
  Byte Packing 4 : xpcutilitieslib/Byte Packing   MaskPackedDataType=int16  MaskUnpackedDataTypes={'uint8'}  MaskAlignment=2
  Degree translation : MATLAB Function  TreatAsAtomicUnit=on
  Gain1 : Gain  Gain=0.01  OutDataTypeStr=double
  Gain4 : Gain  Gain=0.01  OutDataTypeStr=double
  Gain7 : Gain  Gain=0.01  OutDataTypeStr=double
  Mux1 : Mux  Inputs=3
  Selector2 : Selector  InputPortWidth=54  IndexOptions=Index vector (dialog)  Indices=[49 50]  OutputSizes=1
  Selector3 : Selector  InputPortWidth=54  IndexOptions=Index vector (dialog)  Indices=[51 52]  OutputSizes=1
  Selector4 : Selector  InputPortWidth=54  IndexOptions=Index vector (dialog)  Indices=[53 54]  OutputSizes=1
  Out1 : Outport
  wires:
  Gain7/1 -> Degree translation/1(u)
  Byte Packing 3/1 -> Gain4/1
  In1/1 -> Selector2/1, Selector3/1, Selector4/1
  Gain1/1 -> Mux1/1
  Selector3/1 -> Byte Packing 3/1
  Mux1/1 -> Out1/1
  Selector2/1 -> Byte Packing 2/1
  Byte Packing 2/1 -> Gain1/1
  Byte Packing 4/1 -> Gain7/1
  Gain4/1 -> Mux1/2
  Selector4/1 -> Byte Packing 4/1
  Degree translation/1(out) -> Mux1/3

== matlab function Pub_Sensor_20180704/Communication Interface/MATLAB Function4 ==
  data: u input; y output
function y  = fcn(u)
%#codegen
persistent offset
deg = u;
if isempty(offset)
    if u ~= 0
        offset = u;
    end
else
    deg = u - offset;

    if deg <= -180
        deg = 180 + (deg + 180);
    end
    if deg>= 180
        deg = -180 + (deg - 180);
    end
end

y = deg;

== matlab function Pub_Sensor_20180704/Communication Interface/velo逆変換/MATLAB Function ==
  data: velo input; y output; angle input
function y = fcn(velo, angle)
%#codegen

R = [cosd(-angle), -sind(-angle) 0;
    sind(-angle), cosd(-angle) 0;
    0, 0, 1;];

y = R * velo;

== stateflow chart Pub_Sensor_20180704/I//O_Depth/cmDepth ==
  state send
    en:send_q
    state send_q [function]
  state recieve
    entry: data = recieve_data();
    state data = recieve_data [function]
  (default) -> send
  recieve -> send
  send -> recieve
  data: data function_output int16 size=1; data output
  events: event input EITHER_EDGE_EVENT

== matlab function Pub_Sensor_20180704/Communication Interface/bin2data2/Subsystem3/Degree translation ==
  data: u input; out output
function out = fcn(u)
%#codegen
if u > 180 
   out = u - 360;
elseif u < -180
   out = u + 360;
else
   out= u;
end
end

== matlab function Pub_Sensor_20180704/Communication Interface/bin2data2/エラーなら１ (-32768)， それ以外なら0 ==
  data: u input; y output
function y = fcn(u)
%#codegen
if u == -32768
    y = 1;
else
    y = 0;
end

== stateflow chart Pub_Sensor_20180704/I//O_DVL/cm2TRAX2 ==
  state send
    en : send_q
    state send_q [function]
  state recieve
    entry: data = recieve_data();
    state data = recieve_data [function]
  (default) -> send
  recieve -> send
  send -> recieve
  data: data function_output uint8 size=54; data output
  events: event input EITHER_EDGE_EVENT

== matlab function Pub_Sensor_20180704/Communication Interface2/MATLAB Function1 ==
  data: u input; y output
function y  = fcn(u)
%#codegen
persistent offset
deg = u;
if isempty(offset)
    if u ~= 0
        offset = u;
    end
else
    deg = u - offset;

    if deg <= -180
        deg = 180 + (deg + 180);
    end
    if deg>= 180
        deg = -180 + (deg - 180);
    end
end

y = deg;

== matlab function Pub_Sensor_20180704/Communication Interface2/MATLAB Function2 ==
  data: u input; y output
function y  = fcn(u)
%#codegen
persistent offset
deg = u;
if isempty(offset)
    if u ~= 0
        offset = u;
    end
else
    deg = u - offset;

    if deg <= -180
        deg = 180 + (deg + 180);
    end
    if deg>= 180
        deg = -180 + (deg - 180);
    end
end

y = deg;

== matlab function Pub_Sensor_20180704/Communication Interface2/MATLAB Function3 ==
  data: u input; y output
function y  = fcn(u)
%#codegen
persistent offset
deg = u;
if isempty(offset)
    if u ~= 0
        offset = u;
    end
else
    deg = u - offset;

    if deg <= -180
        deg = 180 + (deg + 180);
    end
    if deg>= 180
        deg = -180 + (deg - 180);
    end
end

y = deg;

== stateflow chart Pub_Sensor_20180704/I//O_Gyro/cmGyro ==
  state send
    en:send_q
    state send_q [function]
  state recieve
    entry: data = recieve_data();
    state data = recieve_data [function]
  (default) -> send
  recieve -> send
  send -> recieve
  data: data function_output uint8 size=12; data output
  events: event input EITHER_EDGE_EVENT

== matlab function Pub_Sensor_20180704/座標変換 ==
  data: velo_local input; velo_global output; yaw_angle input
function velo_global = fcn(velo_local, yaw_angle)
%#codegen
R = [cosd(yaw_angle), -sind(yaw_angle);
    sind(yaw_angle), cosd(yaw_angle)];
velo_global = R * velo_local;
